simulink model "Predfiltri"  (R2013b)
settings: Solver=ode45  StartTime=0.0  StopTime=10.0  RelTol=1e-3
libraries: dsparch4 x1
settings Model: Creator=M-Pc  LastModifiedBy=M-Pc

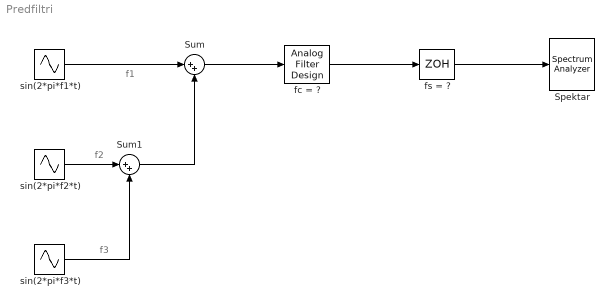
== system Predfiltri ==
  note: f3
  note: f2
  note: f1
  Spektar : SpectrumAnalyzer
      settings: CopyFcn=scopeextensions.ScopeBlock.onCoreBlockCopy(gcbh);  DeleteFcn=scopeextensions.ScopeBlock.callback(gcbh, 'onBlockDelete');  PreSaveFcn=scopeextensions.ScopeBlock.callback(gcbh, 'onModelSave');  NameChangeFcn=scopeextensions.ScopeBlock.callback(gcbh, 'onBlockRename');  DestroyFcn=scopeextensions.ScopeBlock.onBlockDestroy(gcbh)  CloseFcn=scopeextensions.ScopeBlock.callback(gcbh, 'onBlockClose');  PreDeleteFcn=scopeextensions.ScopeBlock.callback(gcbh, 'onBlockPreDelete');
  Sum : Sum  Inputs=|++
  Sum1 : Sum  Inputs=|++
  fc = ? : dsparch4/Analog Filter Design  method=Butterworth  filttype=Lowpass  N=8  Wlo=2*pi*200  Whi=2*pi*180  Rp=2  Rs=40
  fs = ? : ZeroOrderHold  SampleTime=0.0004
  sin(2*pi*f1*t) : Sin  Frequency=2*pi*100  SampleTime=0
  sin(2*pi*f2*t) : Sin  Frequency=2*pi*160  SampleTime=0
  "sin(2*pi*f3*t) " : Sin  Frequency=2*pi*1000  SampleTime=0
  wires:
  sin(2*pi*f1*t)/1 -> Sum/1
  Sum/1 -> fc = ?/1
  fc = ?/1 -> fs = ?/1
  fs = ?/1 -> Spektar/1
  sin(2*pi*f2*t)/1 -> Sum1/1
  "sin(2*pi*f3*t) "/1 -> Sum1/2
  Sum1/1 -> Sum/2
